simulink model "Tractor_Trailer_Platoon"  (Simulink 8.5)
settings: Solver=ode45  StartTime=0.0  StopTime=20  RelTol=1e-3
libraries: Solver_SF x3
settings Model: Creator=elowe  LastModifiedBy=mkhan  CovHtmlReporting=off  CovSFcnEnable=off
settings DebuggingCC: SolverPrmCheckMsg=warning  FcnCallInpInsideContextMsg=EnableAllAsError
settings GRTTargetCC: CombineOutputUpdateFcns=on  GRTInterface=off

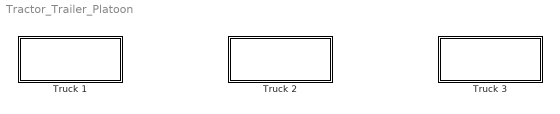
== system Tractor_Trailer_Platoon ==
  Truck 1 : Subsystem
  Truck 2 : Subsystem
  Truck 3 : Subsystem

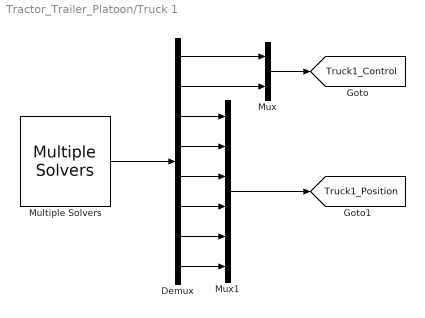
== system Tractor_Trailer_Platoon/Truck 1 ==
  Demux : Demux  Outputs=8
  Multiple Solvers : Solver_SF/Multiple Solvers  Priority=1  iVehicle=1  SIMFILE=D:\product_dev\trunk\Image\TruckSim\Core\TruckSim_Data\Extensions\Simulink\Parallel_Solver\simfile1.sim  Run_RTs=off  vs_state_ind=Run  StopMode_ind=Vehicle Model  vs_scx=on
  Mux : Mux  Inputs=2
  Mux1 : Mux  Inputs=6
  tag scope: Truck1_Control=global, Truck1_Position=global
  wires:
  Multiple Solvers/1 -> Demux/1
  Demux/1 -> Mux/1
  Demux/2 -> Mux/2
  Mux/1 -> [Truck1_Control]
  Mux1/1 -> [Truck1_Position]
  Demux/3 -> Mux1/1
  Demux/4 -> Mux1/2
  Demux/5 -> Mux1/3
  Demux/6 -> Mux1/4
  Demux/7 -> Mux1/5
  Demux/8 -> Mux1/6

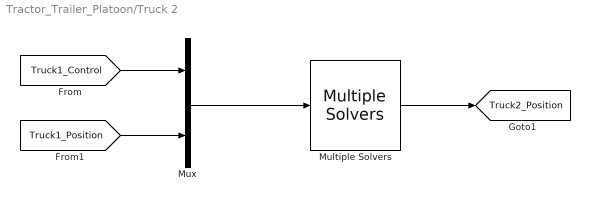
== system Tractor_Trailer_Platoon/Truck 2 ==
  Multiple Solvers : Solver_SF/Multiple Solvers  Priority=1  iVehicle=2  SIMFILE=D:\product_dev\trunk\Image\TruckSim\Core\TruckSim_Data\Extensions\Simulink\Parallel_Solver\simfile2.sim  Run_RTs=off  vs_state_ind=Run  StopMode_ind=Vehicle Model  vs_scx=on
  Mux : Mux  Inputs=2
  tag scope: Truck2_Position=global
  wires:
  Multiple Solvers/1 -> [Truck2_Position]
  [Truck1_Control] -> Mux/1
  Mux/1 -> Multiple Solvers/1
  [Truck1_Position] -> Mux/2

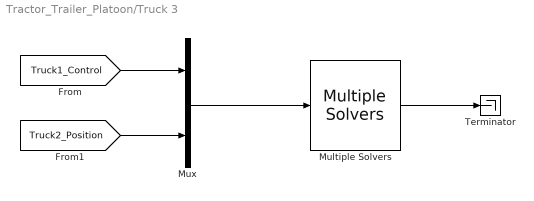
== system Tractor_Trailer_Platoon/Truck 3 ==
  Multiple Solvers : Solver_SF/Multiple Solvers  Priority=1  iVehicle=3  SIMFILE=D:\product_dev\trunk\Image\TruckSim\Core\TruckSim_Data\Extensions\Simulink\Parallel_Solver\simfile3.sim  Run_RTs=off  vs_state_ind=Run  StopMode_ind=Vehicle Model  vs_scx=on
  Mux : Mux  Inputs=2
  Terminator : Terminator
  wires:
  Multiple Solvers/1 -> Terminator/1
  [Truck1_Control] -> Mux/1
  Mux/1 -> Multiple Solvers/1
  [Truck2_Position] -> Mux/2
